simulink model "spindle_test_ramp"  (Simulink 7.6)
settings: Solver=ode4  StartTime=0.0  StopTime=3  FixedStep=0.001  RelTol=1e-3
settings Model: Creator=admin  LastModifiedBy=boshuo
settings DebuggingCC: StrictBusMsg=Warning

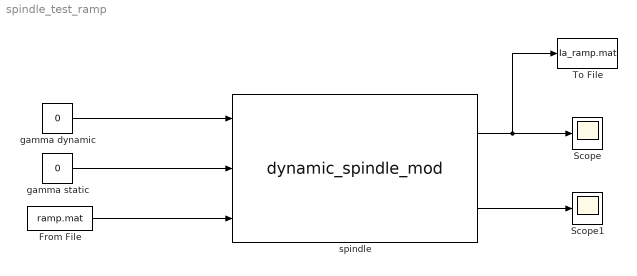
== system spindle_test_ramp ==
  From File : FromFile  FileName=ramp.mat  SampleTime=0
  Scope : Scope
  Scope1 : Scope
  To File : ToFile  Filename=Ia_ramp.mat  MatrixName=firing_output  SaveFormat=Timeseries
  gamma dynamic : Constant  Value=0
  gamma static : Constant  Value=0
  spindle : S-Function  FunctionName=dynamic_spindle_mod  Parameters=[10.4649 10.4649 10.4649] [0.1127 0.1623 0.1623] [0.0605 0.0822 0.0822] [0.2356 -0.046 -0.069] [0 0 0] [0.0289 0.0636 0.0954] [1 0.7 0.7] [1 0.92 0.92] [20000 10000 10000] [20000 7250 7250] [0.3 0.3 0.3] [0.46 0.46 0.46] [0.04 0.04 0.04] [0.76 0.76 0.76] [1 0.04 0.04] [0.192 0.185 0.0001] [0.0002 0.0002 0.0002] [1 0.5 1] [1]  EnableBusSupport=off
      mask Display:
      | port_label('input', 1, 'gamma dynamic');
      | port_label('input', 2, 'gamma static');
      | port_label('input', 3, 'Lce(L0)');
      | port_label('output',1,'Ia');
      | port_label('output',2,'II');
      | disp('Muscle Spindle \n(S-Function)')
  wires:
  From File/1 -> spindle/3
  spindle/1 -> Scope/1, To File/1
  spindle/2 -> Scope1/1
  gamma dynamic/1 -> spindle/1
  gamma static/1 -> spindle/2
